simulink model "MIT_NORMALIZADO"  (Simulink 5.0)
settings: Solver=ode45  StartTime=0.0  StopTime=150  RelTol=1e-3
undefined symbols (not defined in the file): a1, a2, alfa, am, Gama
settings Model: LastModifiedBy=Administrador

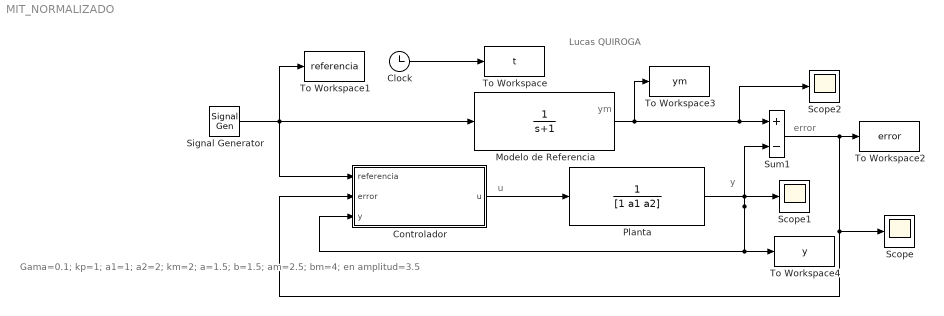
== system MIT_NORMALIZADO ==
  note: y
  note: ym
  note: u
  note: error
  note: Gama=0.1;
      | kp=1;
      | a1=1;
      | a2=2;
      |  km=2;
      | a=1.5;
      | b=1.5;
      | am=2.5;
      | bm=4;
      | en amplitud=3.5
  note: Lucas QUIROGA
  Clock : Clock
  Controlador : Subsystem
  Modelo de Referencia : TransferFcn  Denominator=[1 1]
  Planta : TransferFcn  Denominator=[1 a1 a2]
  Scope : Scope
  Scope1 : Scope
  Scope2 : Scope
      settings: SaveName=ScopeData2
  Signal Generator : SignalGenerator  WaveForm=square  Amplitude=3.5  Frequency=0.05
  Sum1 : Sum  Inputs=+-  SaturateOnIntegerOverflow=on
  To Workspace : ToWorkspace  VariableName=t  SampleTime=-1  SaveFormat=Array
  To Workspace1 : ToWorkspace  VariableName=referencia  SampleTime=-1  SaveFormat=Array
  To Workspace2 : ToWorkspace  VariableName=error  SampleTime=-1  SaveFormat=Array
  To Workspace3 : ToWorkspace  VariableName=ym  SampleTime=-1  SaveFormat=Array
  To Workspace4 : ToWorkspace  VariableName=y  SampleTime=-1  SaveFormat=Array
  wires:
  Controlador/1(u) -> Planta/1
  Signal Generator/1 -> Controlador/1(referencia), To Workspace1/1, Modelo de Referencia/1
  Modelo de Referencia/1 -> To Workspace3/1, Sum1/1, Scope2/1
  Sum1/1 -> To Workspace2/1, Controlador/2(error), Scope/1
  Clock/1 -> To Workspace/1
  Planta/1 -> Scope1/1, To Workspace4/1, Controlador/3(y), Sum1/2

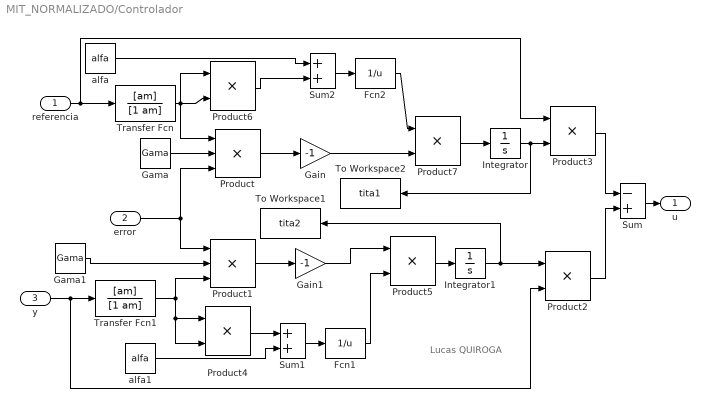
== system MIT_NORMALIZADO/Controlador ==
  note: Lucas QUIROGA
  referencia : Inport
  error : Inport  Port=2
  y : Inport  Port=3
  Fcn1 : Fcn  Expr=1/u
  Fcn2 : Fcn  Expr=1/u
  Gain : Gain  Gain=-1  SaturateOnIntegerOverflow=on
  Gain1 : Gain  Gain=-1  SaturateOnIntegerOverflow=on
  Gama : Constant  Value=Gama
  Gama1 : Constant  Value=Gama
  Integrator : Integrator
  Integrator1 : Integrator
  Product : Product  Inputs=3  SaturateOnIntegerOverflow=on
  Product1 : Product  Inputs=3  SaturateOnIntegerOverflow=on
  Product{2..7} (6 alike) : Product  SaturateOnIntegerOverflow=on
  Sum : Sum  Inputs=-+  SaturateOnIntegerOverflow=on
  Sum1 : Sum  SaturateOnIntegerOverflow=on
  Sum2 : Sum  SaturateOnIntegerOverflow=on
  To Workspace1 : ToWorkspace  VariableName=tita2  SampleTime=-1  SaveFormat=Array
  To Workspace2 : ToWorkspace  VariableName=tita1  SampleTime=-1  SaveFormat=Array
  Transfer Fcn : TransferFcn  Numerator=[am]  Denominator=[1 am]
  Transfer Fcn1 : TransferFcn  Numerator=[am]  Denominator=[1 am]
  alfa : Constant  Value=alfa
  alfa1 : Constant  Value=alfa
  u : Outport
  wires:
  Product/1 -> Gain/1
  Transfer Fcn/1 -> Product/1, Product6/2, Product6/1
  Integrator/1 -> Product3/2, To Workspace2/1
  Product1/1 -> Gain1/1
  Integrator1/1 -> To Workspace1/1, Product2/1
  referencia/1 -> Product3/1, Transfer Fcn/1
  y/1 -> Product2/2, Transfer Fcn1/1
  Product2/1 -> Sum/2
  Product3/1 -> Sum/1
  Sum/1 -> u/1
  Gama/1 -> Product/2
  error/1 -> Product/3, Product1/1
  Gama1/1 -> Product1/2
  Transfer Fcn1/1 -> Product1/3, Product4/1, Product4/2
  Product4/1 -> Sum1/1
  alfa1/1 -> Sum1/2
  Sum1/1 -> Fcn1/1
  Product5/1 -> Integrator1/1
  Fcn1/1 -> Product5/2
  Gain1/1 -> Product5/1
  Product6/1 -> Sum2/2
  alfa/1 -> Sum2/1
  Sum2/1 -> Fcn2/1
  Product7/1 -> Integrator/1
  Fcn2/1 -> Product7/1
  Gain/1 -> Product7/2
